simulink library "Simple_lib"  (R2018b)
settings: Solver=ode45  StartTime=0.0  StopTime=10.0  RelTol=1e-3  EnableMultiTasking=on
undefined symbols (not defined in the file or in its folder): Acceptance, beta, C, C_J, C_P, c_wall, dGain, DiscIntNeverNeededParam, Duplex, Electrical_lib, grab, h_fe, i, i3, K_T, Kman, KmanCE, mu_s, n_rev, R_arm, Simplex, systemTs, tau_0, TinIC, Ts, w_0, wallMass, Watch_lib
libraries: $bdroot x407, PlantUtilityBlockset_lib x30, peGeneralControl x22, simulink x11
(part 3 of 14)

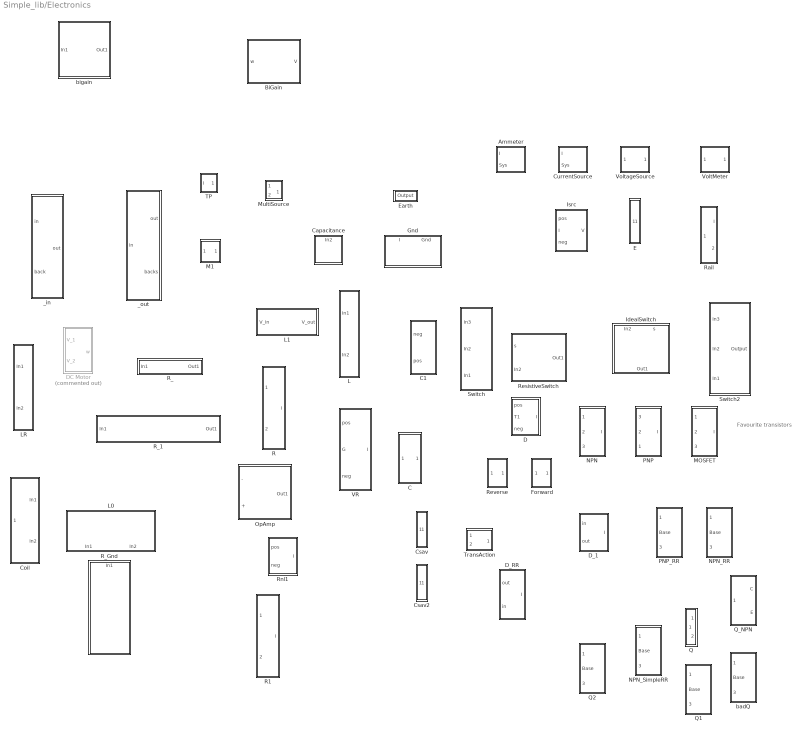
== system Simple_lib/Electronics ==
  note: Favourite transistors
  Ammeter : Subsystem
      mask Display:
      | color('blue')
      | %plot([-1 -.9 -.5 0 .5 .9 1  .9  .5  0 -.5 -.9 -1],      [ 0  .5 .9 1 .9 .5 0 -.5 -.9 -1 -.9 -.5  0]);
      | patch([-1 -.9 -.5 0 .5 .9 1],  [ 0  .5 .9 1 .9 .5 0], [0 0 1]);
      | 
      | %patch([1  .9  .5  0 -.5 -.9 -1], [ 0 -.5 -.9 -1 -.9 -.5  0], [0 0 0]);
      | plot([1  .9  .5  0 -.5 -.9 -1], [ 0 -.5 -.9 -1 -.9 -.5  0]);
      | color('black')
      | disp('A')
      | %plot([0.2 0 -0.2], -[0.7 0.8 0.7])
      | %color('black')
      | %plot([0 0], [0.8 -0.8])
      | 
      | %port_label('output', 1, 'sys ')
      | %color('black')
      | %port_label('output', 2, 'sim ')
  BiGain : Subsystem  mask{k_level=-1, k_flow=-1}
      mask prompts: k_level "Potential Gain"; k_flow "Flow Gain"
      settings: AttributesFormatString="%<k_flow>   %<k_level>"
      mask Display:
      | patch( [0 1 0],[1 0 -1])
      | color('green')
      | plot( [0 -1 0],[1 0 -1])
  C : Subsystem  mask{C=100e-6, Q_0=0}
      mask prompts: C "Capacitance"; Q_0 "Initial Charge (C)"
      settings: AttributesFormatString=%<C>F
      mask Display:
      | %plot([1.0 1.8 1.8 1.0], [0 .1 -.1 0])
      | %patch([-1 -1 -.7 -.7 -1], [-1 1 1 -1 -1])
      | %patch([1 1 .7 .7 1], [-1 1 1 -1 -1])
      | plot([-1 -1], [-1 1])
      | plot([1 1], [-1 1])
      | color('white')
      | plot([-1.1 -1.1], [-1 1])
      | plot([1.1 1.1], [-1 1])
  C1 : Subsystem  mask{C=100e-6}
      mask prompts: C "Capacitance"
      settings: AttributesFormatString=%<C> F
      mask Display:
      | plot([-1 1], [0.5 0.5])
      | plot([-1 1], [-0.5 -0.5])
      | 
      | 
      | color('white')
      | plot([-1 1 1 -1 -1], [-1 -1 1 1 -1])
  Capacitance : Subsystem  mask{C=1e-6}
      mask prompts: C "Capacitance with ground (F)"
      settings: AttributesFormatString=%<C> F
      mask Display:
      | %plot([1.0 1.18 1.18 1.0], [0 .15 -.15 0])
      | plot([0 0],[-1 1])
      | plot([-0.4 -0.4],[-1 1])
      | plot([0.6 0.6], [-0.6 0.6])
      | plot([0.8 0.8],[-0.2 0.2])
      | 
      | plot([-0.4 -1], [0 0])
      | plot([0 0.6],[0 0])
      | 
      | color('white')
      | plot([-1 1 1 -1 -1], [-1 -1 1 1 -1])
  Coil : Subsystem  mask{L=3e-1, R=3e-1, Phi_0=0, L_min=0}
      mask prompts: L "Inductance (H)"; R "Resistance (Ohms)"; Phi_0 "Phi_0 (Vs)"; L_min "L_min (H)"
      settings: AttributesFormatString=|
      | %<L> H
      | %<R> Ohm
      mask Display:
      | %color('black')
      | %plot(   [    0     0.3827     0.7071     0.9239     1.0000     0.9239     0.7071     0.3827     0.0000    -0.3827    -0.7071    -0.9239    -1.0000    -0.9239    -0.7071    -0.3827    -0.0000     0.3827     0.7071     0.9239     1.0000     0.9239     0.7071     0.3827     0.0000    -0.3827    -0.7071    -0.9239    -1.0000    -0.9239    -0.7071    -0.3827    -0.0000     0.3827     0.7071     0.9239     1.0000     0.9239     0.7071     0.3827     0.0000    -0.3827    -0.7071    -0.9239    -1.0000    -0.9239    -0.7071    -0.3827    -0.0000     0.3827     0.7071     0.9239     1.0000     0.9239     0.7071     0.3827     0.0000    -0.3827    -0.7071    -0.9239    -1.0000    -0.9239    -0.7071    -0.3827    -0.0000],   -.5+[-0.0625    -0.0421    -0.0129     0.0230     0.0625     0.1020     0.1379     0.1671     0.1875     0.1984     0.2004     0.1958     0.1875     0.1792     0.1746     0.1766     0.1875     0.2079     0.2371     0.2730     0.3125     0.3520     0.3879     0.4171     0.4375     0.4484     0.4504     0.4458     0.4375     0.4292     0.4246     0.4266     0.4375     0.4579     0.4871     0.5230     0.5625     0.6020     0.6379     0.6671     0.6875     0.6984     0.7004     0.6958     0.6875     0.6792     0.6746     0.6766     0.6875     0.7079     0.7371     0.7730     0.8125     0.8520     0.8879     0.9171     0.9375     0.9484     0.9504     0.9458     0.9375     0.9292     0.9246     0.9266     0.9375])
      | %color('white')
      | %plot([-1 1], [-1 -1])
      | %plot([-1 1], [1 1])
      | color('blue')
      | plot(   .4*[    0     0.3827     0.7071     0.9239     1.0000     0.9239     0.7071     0.3827     0.0000    -0.3827    -0.7071    -0.9239    -1.0000    -0.9239    -0.7071    -0.3827    -0.0000     0.3827     0.7071     0.9239     1.0000     0.9239     0.7071     0.3827     0.0000    -0.3827    -0.7071    -0.9239    -1.0000    -0.9239    -0.7071    -0.3827    -0.0000     0.3827     0.7071     0.9239     1.0000     0.9239     0.7071     0.3827     0.0000    -0.3827    -0.7071    -0.9239    -1.0000    -0.9239    -0.7071    -0.3827    -0.0000     0.3827     0.7071     0.9239     1.0000     0.9239     0.7071     0.3827     0.0000    -0.3827    -0.7071    -0.9239    -1.0000    -0.9239    -0.7071    -0.3827    -0.0000],   -.5+[-0.0625    -0.0421    -0.0129     0.0230     0.0625     0.1020     0.1379     0.1671     0.1875     0.1984     0.2004     0.1958     0.1875     0.1792     0.1746     0.1766     0.1875     0.2079     0.2371     0.2730     0.3125     0.3520     0.3879     0.4171     0.4375     0.4484     0.4504     0.4458     0.4375     0.4292     0.4246     0.4266     0.4375     0.4579     0.4871     0.5230     0.5625     0.6020     0.6379     0.6671     0.6875     0.6984     0.7004     0.6958     0.6875     0.6792     0.6746     0.6766     0.6875     0.7079     0.7371     0.7730     0.8125     0.8520     0.8879     0.9171     0.9375     0.9484     0.9504     0.9458     0.9375     0.9292     0.9246     0.9266     0.9375])
      | plot( [ -.4 .6 -.8 1 ],-.5+[-3:0]/6)
      | plot( [ -.4 .6 -.8 1 ],.5+[0:3]/6)
      | color('white')
      | plot([-1 1 1 -1], [-2 -1 1 2])
  Csav : Subsystem  mask{C=.01, Q_0=0}
      mask prompts: C "Capacitance"; Q_0 "Initial Charge (C)"
      settings: AttributesFormatString=%<C>F
      mask Display:
      | %plot([1.0 1.8 1.8 1.0], [0 .1 -.1 0])
      | %patch([-1 -1 -.7 -.7 -1], [-1 1 1 -1 -1])
      | %patch([1 1 .7 .7 1], [-1 1 1 -1 -1])
      | plot([-1 -1], [-1 1])
      | plot([1 1], [-1 1])
      | color('white')
      | plot([-1.1 -1.1], [-1 1])
      | plot([1.1 1.1], [-1 1])
  Csav2 : Subsystem  mask{C=.01, Q_0=0}
      mask prompts: C "Capacitance"; Q_0 "Initial Charge (C)"
      settings: AttributesFormatString=%<C>F
      mask Display:
      | %plot([1.0 1.8 1.8 1.0], [0 .1 -.1 0])
      | %patch([-1 -1 -.7 -.7 -1], [-1 1 1 -1 -1])
      | %patch([1 1 .7 .7 1], [-1 1 1 -1 -1])
      | plot([-1 -1], [-1 1])
      | plot([1 1], [-1 1])
      | color('white')
      | plot([-1.1 -1.1], [-1 1])
      | plot([1.1 1.1], [-1 1])
  CurrentSource : Subsystem
      mask Display:
      | %plot([-1 -.9 -.5 0 .5 .9 1  .9  .5  0 -.5 -.9 -1],      [ 0  .5 .9 1 .9 .5 0 -.5 -.9 -1 -.9 -.5  0]);
      | 
      | color('blue')
      | %plot([-1 -.9 -.5 0 .5 .9 1  .9  .5  0 -.5 -.9 -1],      [ 0  .5 .9 1 .9 .5 0 -.5 -.9 -1 -.9 -.5  0]);
      | patch([1  .9  .5  0 -.5 -.9 -1],      [ 0 -.5 -.9 -1 -.9 -.5  0], [0 0 1]);
      | 
      | 
      | color('black')
      | plot([-1 -.9 -.5 0 .5 .9 1],      [ 0  .5 .9 1 .9 .5 0]);
      | plot([0 0], [0.8 0])
      | color('white')
      | plot([0 0], [0 -0.8])
      | plot([0.2 0 -0.2], -[0.7 0.8 0.7])
  D : Subsystem  mask{I_S=1e-12, n=2, T_def=300}
      mask prompts: T_def "Default Temp (K)"
      mask Display:
      | %plot( [ -1 0 0 ],[-1 -1 -0.3 ])
      | %plot( [ 0 0 -1],[ 0.3 1 1])
      | plot( [ -1 1],-[1 1]*1.3)
      | plot([-1 1 0 -1],[1 1 -1 1]*1.3)
      | color('white')
      | plot([-1 1], [-2 -2])
      | plot([-1 1], [2 2])
      | %port_label('input', 1, '1')
  DC Motor : Subsystem  Commented=on  mask{k_flow=1, J_mot=1e-3, R_arm=2.0}
      mask prompts: k_flow "Torque constant (Nm/A)"; J_mot "Intertia  (kgm^2)"; R_arm "Armature resistance (Ohm)"
      mask Display:
      | %color('black')
      | %plot( [ -1 0  ],[-1 -1 ])
      | %plot( [ -1 0 ],[ 1 1])
      | 
      | plot([-1 -.9 -.5 0 .5 .9 1  .9  .5  0 -.5 -.9 -1],      [ 0  .5 .9 1 .9 .5 0 -.5 -.9 -1 -.9 -.5  0]);
      | %patch([0 1 1 0 0]-.5,[0 0 1 1 0]*.5-1.5,[0,0,1])
      | %patch([0 1 1 0 0]-.5,[0 0 1 1 0]*.5+1,[0,0,1])
      | color('blue')
      | plot([0 1 1 0 0]-.5,[0 0 1 1 0]*.5-1.5)
      | plot([0 1 1 0 0]-.5,[0 0 1 1 0]*.5+1)
      | %port_label('input', 1, '+')
      | %port_label('input', 2, '-')
      | %port_label('output', 1, 'V')
      | %color('white')
      | %plot([-1 1 1 -1 -1], [-1 -1 1 1 -1]*2)
  D_1 : Subsystem  mask{g_on=0.001, g_off=1e-5, V_drop=1.4}
      mask prompts: g_on "On Conductance (Siemens)"; g_off "Off Conductance (Siemens)"; V_drop "Voltage drop (V)"
      mask Display:
      | %plot( [ -1 0 0 ],[-1 -1 -0.3 ])
      | %plot( [ 0 0 -1],[ 0.3 1 1])
      | plot( [ -1 1],-[1 1]*1.3)
      | patch([-1 1 0 -1],[1 1 -1 1]*1.3)
      | color('white')
      | plot([-1 1], [-2 -2])
      | plot([-1 1], [2 2])
      | %port_label('input', 1, '1')
  D_RR : Subsystem  mask{g=1e-3, V_drop=0.6}
      mask prompts: g "Conductance (Siemens)"; V_drop "Voltage drop (V)"
      mask Display:
      | %plot( [ -1 0 0 ],[-1 -1 -0.3 ])
      | %plot( [ 0 0 -1],[ 0.3 1 1])
      | plot( [ -1 1],-[1 1]*1.3)
      | plot([-1 1 0 -1],[1 1 -1 1]*1.3)
      | color('white')
      | plot([-1 1], [-2 -2])
      | plot([-1 1], [2 2])
      | %port_label('input', 1, '1')
  E : Subsystem  mask{Vbatt=0}
      mask prompts: Vbatt "Voltage (V)"
      settings: AttributesFormatString=EMF: %<Vbatt> V
      mask Display:
      | %color('black')
      | plot([-1 -1], [-0.5 0.5])
      | plot([1 1], [-1 1.0])
      | plot([1 1.1], [0 0])
      | %color('white')
      | %plot([-1 1 1 -1 -1], [-1 -1 1 1 -1])
  Earth : Subsystem
      mask Display:
      | plot([-0.4 -0.4],[-1 1])
      | plot([-0.6 -0.6], [-0.6 0.6])
      | plot([-0.8 -0.8],[-0.2 0.2])
  Forward : Subsystem  mask{V_drop=0.6}
      mask prompts: V_drop "Potential Drop (V)"
      mask Display:
      | patch( [1 1.05 1.05 1],[-1 -1 1 1])
      | patch( [1 0 0],[0 1 -1])
  Gnd : Subsystem
      mask Display:
      | %color('black')
      | %plot([1.0 1.18 1.18 1.0], [0 .15 -.15 0])
      | 
      | plot([-0.1 -0.1],[-.7 .8]+.4)
      | plot([-0.3 -0.3], [-0.6 0.6]+.5)
      | plot([-0.5 -0.5],[-0.2 0.2]+.5)
      | 
      | %plot([-0.1 -0.5],[-1.5 -1.5])
      | 
      | plot([-1 -.9 -.5 0 .5 .9 1  .9  .5  0 -.5 -.9 -1]*.4-.5,      [ 0  .5 .9 1 .9 .5 0 -.5 -.9 -1 -.9 -.5  0]*.9-1.2);
      | plot([-.6 -.3 -.6],[0 .2 .4]-1.3)
      | plot([-.5 -.5],[.1 .3]-1.3)
      | %fprintf('A')
      | %disp('A')
      | %color('white')
      | %plot([-1 1 1 -1 -1], [-1 -1 1 1 -1])
  IdealSwitch : Subsystem
      mask Display:
      | %color('black')
      | %plot([1.0 1.18 1.18 1.0], [0 .2 -.2 0])
      | plot([-1 -0.5], [-0.66 -0.35])
      | plot([-1.0 -0.5]+.3, [-0.66 -0.35]+.5)
      | plot([-.75 -0.5]+.6, [-0.5 -0.35]+.35)
      | 
      | plot([0.1 1], [0 0])
      | plot([-1 -0.5], [0.65 0])
      | color('white')
      | plot([-1 1 1 -1 -1], [-1 -1 1 1 -1])
  Isrc : Subsystem
      mask Display:
      | plot( [ .2 0 -.2],[ -0.4 -.5 -.4])
      | plot( [ 0 0 ],[-1 1]*.5)
      | plot([-1 0 1 0 -1],[0 0.7 0 -0.7 0])
      | port_label('input', 1, '+')
      | port_label('input', 3, '-')
      | color('black')
      | port_label('output', 1, 'V ')
      | port_label('input', 2, ' I')
      | 
      | 
      | color('white')
      | plot([-1 1],[-1 -1])
      | plot([-1 1],[1 1])
  L : Subsystem  mask{L=.1, V_0=0}
      mask prompts: L "Inductance (H)"; V_0 "Initial field"
      settings: AttributesFormatString=|
      | %<L> H
      | %<V_0>
      mask Display:
      | %color('black')
      | plot(   [    0     0.3827     0.7071     0.9239     1.0000     0.9239     0.7071     0.3827     0.0000    -0.3827    -0.7071    -0.9239    -1.0000    -0.9239    -0.7071    -0.3827    -0.0000     0.3827     0.7071     0.9239     1.0000     0.9239     0.7071     0.3827     0.0000    -0.3827    -0.7071    -0.9239    -1.0000    -0.9239    -0.7071    -0.3827    -0.0000     0.3827     0.7071     0.9239     1.0000     0.9239     0.7071     0.3827     0.0000    -0.3827    -0.7071    -0.9239    -1.0000    -0.9239    -0.7071    -0.3827    -0.0000     0.3827     0.7071     0.9239     1.0000     0.9239     0.7071     0.3827     0.0000    -0.3827    -0.7071    -0.9239    -1.0000    -0.9239    -0.7071    -0.3827    -0.0000],   -.5+[-0.0625    -0.0421    -0.0129     0.0230     0.0625     0.1020     0.1379     0.1671     0.1875     0.1984     0.2004     0.1958     0.1875     0.1792     0.1746     0.1766     0.1875     0.2079     0.2371     0.2730     0.3125     0.3520     0.3879     0.4171     0.4375     0.4484     0.4504     0.4458     0.4375     0.4292     0.4246     0.4266     0.4375     0.4579     0.4871     0.5230     0.5625     0.6020     0.6379     0.6671     0.6875     0.6984     0.7004     0.6958     0.6875     0.6792     0.6746     0.6766     0.6875     0.7079     0.7371     0.7730     0.8125     0.8520     0.8879     0.9171     0.9375     0.9484     0.9504     0.9458     0.9375     0.9292     0.9246     0.9266     0.9375])
      | color('white')
      | plot([-1 1], [-1 -1])
      | plot([-1 1], [1 1])
  L0 : Subsystem  mask{L=.1, R=1e3}
      mask prompts: L "Inductance (H)"; R "Resistance (Ohms)"
      settings: AttributesFormatString=|
      | %<L> H
      | %<R> Ohm
      mask Display:
      | %color('black')
      | plot(   [    0     0.3827     0.7071     0.9239     1.0000     0.9239     0.7071     0.3827     0.0000    -0.3827    -0.7071    -0.9239    -1.0000    -0.9239    -0.7071    -0.3827    -0.0000     0.3827     0.7071     0.9239     1.0000     0.9239     0.7071     0.3827     0.0000    -0.3827    -0.7071    -0.9239    -1.0000    -0.9239    -0.7071    -0.3827    -0.0000     0.3827     0.7071     0.9239     1.0000     0.9239     0.7071     0.3827     0.0000    -0.3827    -0.7071    -0.9239    -1.0000    -0.9239    -0.7071    -0.3827    -0.0000     0.3827     0.7071     0.9239     1.0000     0.9239     0.7071     0.3827     0.0000    -0.3827    -0.7071    -0.9239    -1.0000    -0.9239    -0.7071    -0.3827    -0.0000],   -.5+[-0.0625    -0.0421    -0.0129     0.0230     0.0625     0.1020     0.1379     0.1671     0.1875     0.1984     0.2004     0.1958     0.1875     0.1792     0.1746     0.1766     0.1875     0.2079     0.2371     0.2730     0.3125     0.3520     0.3879     0.4171     0.4375     0.4484     0.4504     0.4458     0.4375     0.4292     0.4246     0.4266     0.4375     0.4579     0.4871     0.5230     0.5625     0.6020     0.6379     0.6671     0.6875     0.6984     0.7004     0.6958     0.6875     0.6792     0.6746     0.6766     0.6875     0.7079     0.7371     0.7730     0.8125     0.8520     0.8879     0.9171     0.9375     0.9484     0.9504     0.9458     0.9375     0.9292     0.9246     0.9266     0.9375])
      | color('white')
      | plot([-1 1], [-1 -1])
      | plot([-1 1], [1 1])
  L1 : Subsystem  mask{L=1, R=0}
      mask prompts: L "Inductance (H)"; R "Resistance (Ohms)"
      settings: AttributesFormatString=|
      | %<L> H
      | %<R> Ohm
      mask Display:
      | %color('white')
      | %plot([-1 1 1 -1 -1], [-1 -1 1 1 -1])
      | %color('black')
      | %plot([1.0 1.18 1.18 1.0], [0 .2 -.2 0])
      | plot(-1+2*[-0.0625
      |    -0.0421
      |    -0.0129
      |     0.0230
      |     0.0625
      |     0.1020
      |     0.1379
      |     0.1671
      |     0.1875
      |     0.1984
      |     0.2004
      |     0.1958
      |     0.1875
      |     0.1792
      |     0.1746
      |     0.1766
      |     0.1875
      |     0.2079
      |     0.2371
      |     0.2730
      |     0.3125
      |     0.3520
      |     0.3879
      |     0.4171
      |     0.4375
      |     0.4484
      |     0.4504
      |     0.4458
      |     0.4375
      |     0.4292
      |     0.4246
      |     0.4266
      |     0.4375
      |     0.4579
      |     0.4871
      |     0.5230
      |     0.5625
      |     0.6020
      |     0.6379
      |     0.6671
      |     0.6875
      |     0.6984
      |     0.7004
      |     0.6958
      |     0.6875
      |     0.6792
      |     0.6746
      |     0.6766
      |     0.6875
      |     0.7079
      |     0.7371
      |     0.7730
      |     0.8125
      |     0.8520
      |     0.8879
      |     0.9171
      |     0.9375
      |     0.9484
      |     0.9504
      |     0.9458
      |     0.9375
      |     0.9292
      |     0.9246
      |     0.9266
      |     0.9375], [    0
      |     0.3827
      |     0.7071
      |     0.9239
      |     1.0000
      |     0.9239
      |     0.7071
      |     0.3827
      |     0.0000
      |    -0.3827
      |    -0.7071
      |    -0.9239
      |    -1.0000
      |    -0.9239
      |    -0.7071
      |    -0.3827
      |    -0.0000
      |     0.3827
      |     0.7071
      |     0.9239
      |     1.0000
      |     0.9239
      |     0.7071
      |     0.3827
      |     0.0000
      |    -0.3827
      |    -0.7071
      |    -0.9239
      |    -1.0000
      |    -0.9239
      |    -0.7071
      |    -0.3827
      |    -0.0000
      |     0.3827
      |     0.7071
      |     0.9239
      |     1.0000
      |     0.9239
      |     0.7071
      |     0.3827
      |     0.0000
      |    -0.3827
      |    -0.7071
      |    -0.9239
      |    -1.0000
      |    -0.9239
      |    -0.7071
      |    -0.3827
      |    -0.0000
      |     0.3827
      |     0.7071
      |     0.9239
      |     1.0000
      |     0.9239
      |     0.7071
      |     0.3827
      |     0.0000
      |    -0.3827
      |    -0.7071
      |    -0.9239
      |    -1.0000
      |    -0.9239
      |    -0.7071
      |    -0.3827
      |    -0.0000])
  LR : Subsystem  mask{L=1e-6, R=R_arm, Phi_0=0}
      mask prompts: L "Inductance (H)"; R "Resistance (Ohms)"; Phi_0 "Phi_0 (Vs)"
      settings: AttributesFormatString=|
      | %<L> H
      | %<R> Ohm
      mask Display:
      | %color('black')
      | %plot(   [    0     0.3827     0.7071     0.9239     1.0000     0.9239     0.7071     0.3827     0.0000    -0.3827    -0.7071    -0.9239    -1.0000    -0.9239    -0.7071    -0.3827    -0.0000     0.3827     0.7071     0.9239     1.0000     0.9239     0.7071     0.3827     0.0000    -0.3827    -0.7071    -0.9239    -1.0000    -0.9239    -0.7071    -0.3827    -0.0000     0.3827     0.7071     0.9239     1.0000     0.9239     0.7071     0.3827     0.0000    -0.3827    -0.7071    -0.9239    -1.0000    -0.9239    -0.7071    -0.3827    -0.0000     0.3827     0.7071     0.9239     1.0000     0.9239     0.7071     0.3827     0.0000    -0.3827    -0.7071    -0.9239    -1.0000    -0.9239    -0.7071    -0.3827    -0.0000],   -.5+[-0.0625    -0.0421    -0.0129     0.0230     0.0625     0.1020     0.1379     0.1671     0.1875     0.1984     0.2004     0.1958     0.1875     0.1792     0.1746     0.1766     0.1875     0.2079     0.2371     0.2730     0.3125     0.3520     0.3879     0.4171     0.4375     0.4484     0.4504     0.4458     0.4375     0.4292     0.4246     0.4266     0.4375     0.4579     0.4871     0.5230     0.5625     0.6020     0.6379     0.6671     0.6875     0.6984     0.7004     0.6958     0.6875     0.6792     0.6746     0.6766     0.6875     0.7079     0.7371     0.7730     0.8125     0.8520     0.8879     0.9171     0.9375     0.9484     0.9504     0.9458     0.9375     0.9292     0.9246     0.9266     0.9375])
      | %color('white')
      | %plot([-1 1], [-1 -1])
      | %plot([-1 1], [1 1])
      | 
      | plot(   .4*[    0     0.3827     0.7071     0.9239     1.0000     0.9239     0.7071     0.3827     0.0000    -0.3827    -0.7071    -0.9239    -1.0000    -0.9239    -0.7071    -0.3827    -0.0000     0.3827     0.7071     0.9239     1.0000     0.9239     0.7071     0.3827     0.0000    -0.3827    -0.7071    -0.9239    -1.0000    -0.9239    -0.7071    -0.3827    -0.0000     0.3827     0.7071     0.9239     1.0000     0.9239     0.7071     0.3827     0.0000    -0.3827    -0.7071    -0.9239    -1.0000    -0.9239    -0.7071    -0.3827    -0.0000     0.3827     0.7071     0.9239     1.0000     0.9239     0.7071     0.3827     0.0000    -0.3827    -0.7071    -0.9239    -1.0000    -0.9239    -0.7071    -0.3827    -0.0000],   -.5+[-0.0625    -0.0421    -0.0129     0.0230     0.0625     0.1020     0.1379     0.1671     0.1875     0.1984     0.2004     0.1958     0.1875     0.1792     0.1746     0.1766     0.1875     0.2079     0.2371     0.2730     0.3125     0.3520     0.3879     0.4171     0.4375     0.4484     0.4504     0.4458     0.4375     0.4292     0.4246     0.4266     0.4375     0.4579     0.4871     0.5230     0.5625     0.6020     0.6379     0.6671     0.6875     0.6984     0.7004     0.6958     0.6875     0.6792     0.6746     0.6766     0.6875     0.7079     0.7371     0.7730     0.8125     0.8520     0.8879     0.9171     0.9375     0.9484     0.9504     0.9458     0.9375     0.9292     0.9246     0.9266     0.9375])
      | plot( [ -.4 .6 -.8 1 ],-.5+[-3:0]/6)
      | plot( [ -.4 .6 -.8 1 ],.5+[0:3]/6)
      | color('white')
      | plot([-1 1 1 -1], [-2 -1 1 2])
  M1 : Subsystem
      mask Display:
      | plot([-1 -.9 -.5 0 .5 .9 1  .9  .5  0 -.5 -.9 -1],      [ 0  .5 .9 1 .9 .5 0 -.5 -.9 -1 -.9 -.5  0]);
      | disp('M')
  MOSFET : Subsystem  mask{V_T=1.7, k=5}
      mask Display:
      | patch([0 0 0.05 0.05]-0.2,[-.3 .3 .3 -.3])
      | patch([0 0 0.1 0.1],[-1 1 1 -1])
      | %patch([0 0 0.1 0.1],[-1 -.6 -.6 -1],[.9 .5 .1])
      | 
      | plot([0 1],[0.66 0.66])
      | plot([0 1],[0 0])
      | plot([0 1],[-0.66 -0.66])
      | plot([1 1],[-0.66 0])
      | patch([0.1 .3 .3],[0 .1 -0.1])
  MultiSource : Subsystem  mask{V_0=inf, slew_rate=inf, conserved_quantity_name=Q, energy_name=E}
      mask prompts: V_0 "Iniitial Potential (V)"; slew_rate "Max +/- slew rate (V/s)"; conserved_quantity_name "Conserved quantity name"; energy_name "Energy name"
      mask init:
      | init_lump
      mask Display:
      | plot([-1 -.9 -.5 0 .5 .9 1  .9  .5  0 -.5 -.9 -1],      [ 0  .5 .9 1 .9 .5 0 -.5 -.9 -1 -.9 -.5  0]);
      | %disp(get(gcbh,'Name'))
  NPN : Subsystem  mask{alpha_F=0.98, alpha_R=0.9, n=1, I_S=1e-12, T_def=300}
      mask prompts: n "Emission Coefficient"; T_def "Default temp (when input==0) (K)"
      mask Display:
      | patch([0 0 0.1 0.1],[-1 1 1 -1])
      | %patch([0 0 0.1 0.1],[-1 -.7 -.7 -1],[.9 .5 .1])
      | 
      | plot([0 1],[0.25 1])
      | plot([0 1],[-0.25 -1])
      | 
      | patch([.8 1 1],[-1 -1 -0.8])
  NPN_RR : Subsystem  mask{alpha_F=0.98, alpha_R=0.9}
      mask Display:
      | patch([0 0 0.1 0.1],[-1 1 1 -1])
      | %patch([0 0 0.1 0.1],[-1 -.7 -.7 -1],[.9 .5 .1])
      | 
      | plot([0 1],[0.25 1])
      | plot([0 1],[-0.25 -1])
      | 
      | patch([.8 1 1],[-1 -1 -0.8])
  NPN_SimpleRR : Subsystem  mask{alpha_F=0.98, alpha_R=0.9}
      mask Display:
      | patch([0 0 0.1 0.1],[-1 1 1 -1])
      | %patch([0 0 0.1 0.1],[-1 -.7 -.7 -1],[.9 .5 .1])
      | 
      | plot([0 1],[0.25 1])
      | plot([0 1],[-0.25 -1])
      | 
      | patch([.8 1 1],[-1 -1 -0.8])
  OpAmp : Subsystem  mask{K_op=6}
      mask prompts: K_op "K_op (-)"
      mask Display:
      | %patch( [1 1.05 1.05 1],[-1 -1 1 1])
      | plot( [1 0 0 1],[0 1 -1 0])
      | port_label('input', 1, '+')
      | port_label('input', 2, '-')
  PNP : Subsystem  mask{alpha_F=0.98, alpha_R=0.9}
      mask Display:
      | patch([0 0 0.1 0.1],[-1 1 1 -1])
      | %patch([0 0 0.1 0.1],[-1 -.7 -.7 -1],[.9 .5 .1])
      | 
      | plot([0 1],[0.25 1])
      | plot([0 1],[-0.25 -1])
      | 
      | patch([.1 .35 .2],[-0.25 -0.35 -0.5])
  PNP_RR : Subsystem  mask{alpha_F=0.98, alpha_R=0.9}
      mask Display:
      | patch([0 0 0.1 0.1],[-1 1 1 -1])
      | %patch([0 0 0.1 0.1],[-1 -.7 -.7 -1],[.9 .5 .1])
      | 
      | plot([0 1],[0.25 1])
      | plot([0 1],[-0.25 -1])
      | 
      | patch([.1 .35 .2],[-0.25 -0.35 -0.5])
  Q : Subsystem  mask{alpha_F=0.98, alpha_R=0.9}
      mask Display:
      | patch([1 1 0.9 0.9],[-1 1 1 -1])
      | %patch([0 0 0.1 0.1],[-1 -.7 -.7 -1],[.9 .5 .1])
      | 
      | plot([1 0], [0.05 0.5])
      | plot([1 0], [-0.05 -0.5])
      | 
      | patch([.2 0 0.1], [-.5 -.5 -0.35])
  Q1 : Subsystem  mask{alpha_F=0.98, alpha_R=0.9, g_on=10, g_off=1e-6, V_drop=0.6}
      mask prompts: g_on "diode g on (S)"; g_off "diode g off"; V_drop "diode drop (V)"
      mask Display:
      | patch([0 0 0.1 0.1],[-1 1 1 -1])
      | %patch([0 0 0.1 0.1],[-1 -.7 -.7 -1],[.9 .5 .1])
      | 
      | plot([0 1],[0.25 1])
      | plot([0 1],[-0.25 -1])
      | 
      | patch([.8 1 1],[-1 -1 -0.8])
  Q2 : Subsystem  mask{alpha_F=0.98, alpha_R=0.9, g_on=10, g_off=1e-6, V_drop=0.6}
      mask Display:
      | patch([0 0 0.1 0.1],[-1 1 1 -1])
      | %patch([0 0 0.1 0.1],[-1 -.7 -.7 -1],[.9 .5 .1])
      | 
      | plot([0 1],[0.25 1])
      | plot([0 1],[-0.25 -1])
      | 
      | patch([.1 .35 .2],[-0.25 -0.35 -0.5])
  Q_NPN : Subsystem  mask{alpha_F=0.98, alpha_R=0.1}
      mask Display:
      | patch([0 0 0.1 0.1],0.5*[-1 1 1 -1])
      | %patch([0 0 0.1 0.1],[-1 -.7 -.7 -1],[.9 .5 .1])
      | 
      | plot([0 1],[0.2 0.5])
      | plot([0 1],[-0.2 -0.5])
      | 
      | patch([.8 1 1],[-0.53 -0.53 -0.4])
      | color('white')
      | plot([0 0],[-1 1])
  R : Subsystem  mask{R=100e3}
      mask prompts: R "Resistance (Ohms)"
      settings: AttributesFormatString=%<R> Ohms
      mask Display:
      | plot( [ -1 1 -1 1 -1 1 -1],[-3:3]/6)
      | 
      | port_label('input',1,'+')
      | port_label('input',2,'-')
      | color('white')
      | plot([-1 1 1 -1 -1], [-1 -1 1 1 -1])
  R1 : Subsystem  mask{R=100e3}
      mask prompts: R "Resistance (Ohms)"
      settings: AttributesFormatString=%<R> Ohms
      mask Display:
      | plot( [ -1 1 -1 1 -1 1 -1],[-3:3]/6)
      | 
      | port_label('input',1,'+')
      | port_label('input',2,'-')
      | color('white')
      | plot([-1 1 1 -1 -1], [-1 -1 1 1 -1])
  R_ : Subsystem  mask(Circuit Resistor){Mantissa=1.0, Exponent=3, R=1000}
      mask prompts: Mantissa "Resistance (Ohm)"; Exponent "e"
      mask help: This block contains an Ohmic Resistance, and a test point at its outport.
      mask init:
      | newR = str2num(Mantissa) * 10^Exponent;
      | set(gcbh,'R', num2str(newR))
      settings: AttributesFormatString=%<R> Ohm
      mask Help:
      | Choose one of the standard resistance values or type your own.
      | e means the power of 10 that the chosen resistance value will be multiplied by to make the actual resistance used.
      mask TypeOptions Mantissa: 1.0 | 1.2 | 1.5 | 1.8 | 2.2 | 2.7 | 3.3 | 3.9 | 4.7 | 5.6 | 6.8 | 8.2
      mask DialogControl Exponent Tooltip: Times this power of ten
      mask Display:
      | %color('black')
      | %plot([1.0 1.18 1.18 1.0], [0 .2 -.2 0])
      | plot([-8:8]/8, [0 1 0 -1 0 1 0 -1 0 1 0 -1 0 1 0 -1 0])
      | 
      | color('white')
      | plot([-1 1 1 -1 -1], [-1 -1 1 1 -1])
  R_1 : Subsystem  mask{R=0}
      mask prompts: R "Resistance"
      settings: AttributesFormatString=%<R> Ohm
      mask Display:
      | %color('black')
      | %plot([1.0 1.18 1.18 1.0], [0 .2 -.2 0])
      | plot([-8:8]/8, [0 1 0 -1 0 1 0 -1 0 1 0 -1 0 1 0 -1 0])
      | 
      | color('white')
      | plot([-1 1 1 -1 -1], [-1 -1 1 1 -1])
  R_Gnd : Subsystem  mask{R=15e3}
      mask prompts: R "Resistance"
      settings: AttributesFormatString=%<R> Ohm
      mask Display:
      | %color('black')
      | %plot([1.0 1.18 1.18 1.0], [0 .2 -.2 0])
      | plot([-8:8]/8, [0 1 0 -1 0 1 0 -1 0 1 0 -1 0 1 0 -1 0])
      | 
      | plot([0 0]+2.6, 0.9*[-1 1])
      | plot([0 0]+2.8, 0.75*[-1 1])
      | plot([0 0]+3, 0.5*[-1 1])
      | 
      | plot([1 2.6],[0 0])
      | 
      | color('white')
      | plot([-1 1 1 -1 -1], [-1 -1 1 1 -1])
  Rail : Subsystem  mask{Vcc=12}
      mask prompts: Vcc "Vcc offset  (V)"
      settings: AttributesFormatString=in +%<Vcc> V
      mask Display:
      | %color('black')
      | plot([-.9 -.9], [-0.5 0.5])
      | plot([.9 .9], [-1 1.0])
      | color('white')
      | plot([-1 1 1 -1 -1], [-1 -1 1 1 -1])
  ResistiveSwitch : Subsystem
      mask Display:
      | %color('black')
      | %plot([1.0 1.18 1.18 1.0], [0 .2 -.2 0])
      | plot([-1 -0.5], [-0.66 -0.35])
      | plot([-1.0 -0.5]+.3, [-0.66 -0.35]+.5)
      | plot([-.75 -0.5]+.6, [-0.5 -0.35]+.35)
      | 
      | plot([0.1 1], [0 0])
      | plot([-1 -0.5], [0.65 0])
      | color('white')
      | plot([-1 1 1 -1 -1], [-1 -1 1 1 -1])
  Reverse : Subsystem  mask{V_drop=0}
      mask prompts: V_drop "Potential Drop (V)"
      mask Display:
      | patch( [0 -0.05 -0.05 0],[-1 -1 1 1])
      | patch( [0 1 1],[0 1 -1])
  Rnl1 : Subsystem  mask{I_S=1e-12, n=2, T_def=300}
      mask prompts: T_def "Default Temp (K)"
      mask Display: plot( [ -1.2 0.8 -1 1.2 -1 1.5 -1],[-3:3]/6)
  Switch : Subsystem
      mask Display:
      | %color('black')
      | plot( [ -1 0 0 ], [ 1 1 .3 ]*2/3 )
      | plot( [ -1 0 0 ],-[ 1 1 .3 ]*2/3 )
      | plot( [ -1 -1 ]/2,[ -.3 .3 ]*2/3 )
      | 
      | color('white')
      | plot([-1 1 1 -1 -1], [-1 -1 1 1 -1])
  Switch2 : Subsystem
      mask Display:
      | %color('black')
      | plot( [ -1 0 0 ], [ 1 1 .3 ]*2/3 )
      | plot( [ -1 0 0 ],-[ 1 1 .3 ]*2/3 )
      | plot( [ 0 1 ],[ .2 0 ] )
      | patch( [ 0 .22 0],[ .2 .22 .15] )
      | plot( [ -1 +.7 ],[ 0 0 ] )
      | 
      | color('white')
      | plot([-1 1 1 -1 -1], [-1 -1 1 1 -1])
  TP : Subsystem  mask{V_0=0.0, slew_rate=inf, conserved_quantity_name=Q, energy_name=E}
      mask prompts: V_0 "Iniitial Potential (V)"; slew_rate "Max +/- slew rate (V/s)"; conserved_quantity_name "Conserved quantity name"; energy_name "Energy name"
      mask init:
      | init_lump
      mask Display:
      | plot([-1 -.9 -.5 0 .5 .9 1  .9  .5  0 -.5 -.9 -1],      [ 0  .5 .9 1 .9 .5 0 -.5 -.9 -1 -.9 -.5  0]);
      | %disp(get(gcbh,'Name'))
  TransAction : Subsystem  mask{V_drop=.6}
      mask prompts: V_drop "Potential Drop (V)"
      mask Display:
      | patch( [0 -0.05 -0.05 0],[-1 -1 1 1])
      | patch( [0 1 1],[0 1 -1])
  VR : Subsystem
      mask Display:
      | plot( [ -1 1 -1 1 -1 1 -1],[-3:3]/6)
      | plot( [ 1 -1]*0.8,[-1 1]*0.8)
      | patch([0.6 0.8 0.8],-[0.8 0.8 0.6])
      | color('white')
      | plot([-1 1 1 -1 -1], [-1 -1 1 1 -1])
  VoltMeter : Subsystem
      mask Display:
      | %plot([-1 -.9 -.5 0 .5 .9 1  .9  .5  0 -.5 -.9 -1],      [ 0  .5 .9 1 .9 .5 0 -.5 -.9 -1 -.9 -.5  0]);
      | color('black')
      | plot([0 .5 .9 1  .9  .5  0],      [ 1 .9 .5 0 -.5 -.9 -1]);
      | patch(-[0 .5 .9 1  .9  .5  0],  [ 1 .9 .5 0 -.5 -.9 -1] ,[0 0 1]  );
      | %plot([0 0], [0 -0.8])
      | %plot([0.2 0 -0.2], -[0.7 0.8 0.7])
      | %port_label('output', 1, '+ ')
      | color('black')
      | disp('V')
  VoltageSource : Subsystem
      mask Display:
      | %plot([-1 -.9 -.5 0 .5 .9 1  .9  .5  0 -.5 -.9 -1],      [ 0  .5 .9 1 .9 .5 0 -.5 -.9 -1 -.9 -.5  0]);
      | %plot([0 0], [0 -0.8])
      | %plot([0.2 0 -0.2], -[0.7 0.8 0.7])
      | patch([0 .5 .9 1  .9  .5  0],      [ 1 .9 .5 0 -.5 -.9 -1], [0 0 1]);
      | color('black')
      | plot(-[0 .5 .9 1  .9  .5  0],  [ 1 .9 .5 0 -.5 -.9 -1] );
      | %port_label('input', 1, ' V')
      | color('white')
      | port_label('output', 1, '+ ')
  _in : Subsystem  InitFcn=""  mask{Level=V, Flow=I}
      mask prompts: Level "Level variable name:"; Flow "Flow variable name:"
      mask init:
      | init_in
      mask Display:
      | %% Icon for flow in
      | % Signally design
      | %plot([0 2 2 3], [1 1 0 0])
      | %plot([1 3 2 1 0 2], [0.6 0.6 0.4 0.6 0.4 0.4])
      | %patch([1 3 2],[0.6 0.6 0.4])
      | %plot([0 1 1], [1 1 0.6])
      | %plot([1 1 0], [0.4 -1 -1])
      | 
      | %color('white')
      | %plot([0 3], [2 2])
      | %plot([0 3], [-2 -2])
      | 
      | %% Bolder design
      | %patch( [0 1 -1], [0 1 1])
      | %plot( [-1 1], [1.05 1.05])
      | %patch( [-0.1 -0.1 -1], [0.95 0 0.95])
      | patch( [-0.1 -0.1 -1], [1 0 1])
      | patch( [0.1 0.1 1], [1 0 1])
      | plot( [0.1 1 -1 -0.1], [0 -2 -2 0]*0.5)
      | %patch( [-0.1 0.1 0.1 -0.1], [0 0 1 1], [1 1 1])
      | %patch( [-1 0.1 0.1 -1], [1 1 0.95 0.95], [1 1 1])
      | 
      | %% Size the box
      | color('white')
      | plot( [-1 1], [2 2])
      | plot( [-1 1], -[2 2])
  _out : Subsystem  Tag=Electrical  mask{Level=V, Flow=I}
      mask prompts: Level "Level variable name:"; Flow "Flow variable name:"
      mask init:
      | init_out
      mask Display:
      | % This is a new mask on top of the base mask.
      | % Use "View base mask" link below to see the base mask.
      | % Icon for flow out
      | %% Complex icon
      | %plot([0 1 1], [0 0 0.4])
      | %plot([1 1 3], [0.6 1 1])
      | %plot([1 3 2 1 0 2], [0.6 0.6 0.4 0.6 0.4 0.4])
      | %patch([0 2 1],[0.4 0.4 0.6])
      | %plot([3 2 2], [1 1 0.6])
      | %plot([2.2 2.2], [1 0.6])
      | %plot([1.8 1.8], [1 0.6])
      | %plot([1.6 2.4], [0 0])
      | %plot([2 2], [0.1 -0.1])
      | %plot([2 2], [0.4 0.2])
      | %plot([2 2 3], [-0.2 -1 -1])
      | 
      | %color('white')
      | %plot([0 3], [2 2])
      | %plot([0 3], [-2 -2])
      | 
      | %% Bolder icon
      | plot([-1 0 1], [0 -1 0])
      | %patch([-1 1 0 -1], [1 1 2 1]*1-1)
      | patch([-1 -.2 -.2], [0 0 1])
      | patch([1 .2 .2], [0 0 1])
      | %patch( [-0.1 0.1 0.1 -0.1], [0 0 1 1], [1 1 1])
      | plot(0.2*[-1 1],-0.3*[1  1]+0*1.5)
      | plot([0 0],[-0.15 -0.45]+0*1.5)
      | 
      | 
      | color('white')
      | plot( [-1 1], [2 2])
      | plot( [-1 1], -[2 2])
  badQ : Subsystem  mask{alpha_F=0.98, alpha_R=0.9}
      mask Display:
      | patch([0 0 0.1 0.1],[-1 1 1 -1])
      | %patch([0 0 0.1 0.1],[-1 -.7 -.7 -1],[.9 .5 .1])
      | 
      | plot([0 1],[0.25 1])
      | plot([0 1],[-0.25 -1])
      | 
      | patch([.8 1 1],[-1 -1 -0.8])
  bigain : Subsystem
      mask Display:
      | %patch( [1 1.05 1.05 1],[-1 -1 1 1])
      | patch( [1 0 0],[0 1 -1])
      | plot( [0 1 1],[1 2 0])

== system Simple_lib/Hydraulic ==
  " Heat Exchanger" : Subsystem  AncestorBlock="PlantUtilityBlockset_lib/Hydraulic/ Heat  Exchanger"
      mask Display:
      | color('white');
      | plot([-3 3],[1 1]);
      | plot([-3 3],[-1 -1]);
      | color('black')
      | 
      | plot(2+[ 0 .5 .9 1  .9  .5  0 ], [ 1 .9 .5 0 -.5 -.9 -1 ]);
      | plot(-2-[ 0 .5 .9 1  .9  .5  0 ], [ 1 .9 .5 0 -.5 -.9 -1 ]);
      | 
      | plot([-1.5 -1.5],[-1 1]);
      | plot([1.5 1.5],[-1 1]);
      | 
      | plot([-1.5 1.5],[1.0 1.0]);
      | plot([-1.5 1.5],[0.5 0.5]);
      | plot([-1.5 1.5],[0 0]);
      | plot([-1.5 1.5],[-0.5 -0.5]);
      | plot([-1.5 1.5],[-1.0 -1.0]);
  Accumulator : Subsystem
      mask Display:
      | color('white');
      | plot([-1 1],[1 1]);
      | plot([-1 1],[-1 -1]);
      | color('black')
      | plot([0 0],[-1 1]);
      | plot([-1 -.9 -.5 0 .5 .9 1  .9  .5  0 -.5 -.9 -1],      [ 0  .5 .9 1 .9 .5 0 -.5 -.9 -1 -.9 -.5  0]);
      | plot([0 -0.2 -0.4 -0.6],[-0.25 0.25 -0.25 0.25])
      | plot([1 1.5 1.5 1],[0 -0.25 0.25 0])
  Atmosphere : Subsystem
      mask Display:
      | color('white')
      | plot([-1 1 1 -1 -1], [-1 -1 1 1 -1])
      | 
      | color('black')
      | plot([1.0 1.18 1.18 1.0], [0 .15 -.15 0])
      | 
      | plot([-0.4 -0.4],[-1 1])
      | plot([-0.4 0], [-1 -1])
      | plot([-0.4 0],[1 1])
      | 
      | plot([-0.3 1],[0 0])
  Heat Sink : Subsystem
  Isothermal Accumulator : Subsystem
      mask Display:
      | color('white');
      | plot([-1 1],[1 1]);
      | plot([-1 1],[-1 -1]);
      | color('black')
      | plot([0 0],[-1 1]);
      | plot([-1 -.9 -.5 0 .5 .9 1  .9  .5  0 -.5 -.9 -1],      [ 0  .5 .9 1 .9 .5 0 -.5 -.9 -1 -.9 -.5  0]);
      | plot([0 -0.2 -0.4 -0.6],[-0.25 0.25 -0.25 0.25])
      | plot([1 1.5 1.5 1],[0 -0.25 0.25 0])
  Isothermal Pump : Subsystem
      mask Display:
      | color('white');
      | plot([-1 1],[1 1]);
      | plot([-1 1],[-1 -1]);
      | color('black')
      | 
      | plot([-1 -.9 -.5 0 .5 .9 1  .9  .5  0 -.5 -.9 -1],      [ 0  .5 .9 1 .9 .5 0 -.5 -.9 -1 -.9 -.5  0]);
      | 
      | patch([0 -0.25 0.25 0],[1 .5 .5 1])
      | patch([0 -0.25 0.25 0],-[1 .5 .5 1])
  Isothermal Tank : Subsystem
      mask Display:
      | color('white')
      | plot([-1 1 1 -1 -1], [-1 -1 1 1 -1])
      | 
      | color('black')
      | plot([1.0 1.18 1.18 1.0], [0 .15 -.15 0])
      | 
      | plot([-0.4 -0.4],[-1 1])
      | plot([-0.4 0], [-1 -1])
      | plot([-0.4 0],[1 1])
      | 
      | plot([-0.3 1],[0 0])
  Linear Heat Pipe : Subsystem
      mask Display:
      | plot([-1:0.2:1], [1 .8 .6 .5 .5 .5 .5 .5 .6 .8 1])
      | plot([-1:0.2:1], -[1 .8 .6 .5 .5 .5 .5 .5 .6 .8 1])
  Linear Pipe : Subsystem
      mask Display:
      | plot([-1:0.2:1], [1 .8 .6 .5 .5 .5 .5 .5 .6 .8 1])
      | plot([-1:0.2:1], -[1 .8 .6 .5 .5 .5 .5 .5 .6 .8 1])
  Motor : Subsystem
      mask Display:
      | color('white');
      | plot([-1 1],[1 1]);
      | plot([-1 1],[-1 -1]);
      | color('black')
      | 
      | plot([-1 -.9 -.5 0 .5 .9 1  .9  .5  0 -.5 -.9 -1],      [ 0  .5 .9 1 .9 .5 0 -.5 -.9 -1 -.9 -.5  0]);
      | 
      | text(0,0,'M')
      | plot([1 1.5 1.5 1],[0 -0.25 0.25 0])
  Pressure Meter : Subsystem
      mask Display:
      | color('white')
      | plot([-1 1 1 -1 -1], [-1 -1 1 1 -1])
      | color('black')
      | 
      | plot([-1 -.9 -.5 0 .5 .9 1  .9  .5  0 -.5 -.9 -1], ...
      |     [ 0  .5 .9 1 .9 .5 0 -.5 -.9 -1 -.9 -.5  0]);
      | plot(.7*[-1 1], .7*[-1 1])
      | plot(.7*[-1 1], .7*[1 -1])
      | 
      | %text(0, 0, 'p')
  Pump : Subsystem
      mask Display:
      | color('white');
      | plot([-1 1],[1 1]);
      | plot([-1 1],[-1 -1]);
      | color('black')
      | 
      | plot([-1 -.9 -.5 0 .5 .9 1  .9  .5  0 -.5 -.9 -1],      [ 0  .5 .9 1 .9 .5 0 -.5 -.9 -1 -.9 -.5  0]);
      | 
      | patch([0 -0.25 0.25 0],[1 .5 .5 1])
      | patch([0 -0.25 0.25 0],-[1 .5 .5 1])
  Quadratic Heat Pipe : Subsystem
      mask Display:
      | plot([-1:0.2:1], [1 .7 .5 .4 .35 .32 .35 .4 .5 .7 1])
      | plot([-1:0.2:1], -[1 .7 .5 .4 .35 .32 .35 .4 .5 .7 1])
  Quadratic Pipe : Subsystem
      mask Display:
      | plot([-1:0.2:1], [1 .7 .5 .4 .35 .32 .35 .4 .5 .7 1])
      | plot([-1:0.2:1], -[1 .7 .5 .4 .35 .32 .35 .4 .5 .7 1])
  Tank : Subsystem
      mask Display:
      | color('white')
      | plot([-1 1 1 -1 -1], [-1 -1 1 1 -1])
      | 
      | color('black')
      | plot([1.0 1.18 1.18 1.0], [0 .15 -.15 0])
      | 
      | plot([-0.4 -0.4],[-1 1])
      | plot([-0.4 0], [-1 -1])
      | plot([-0.4 0],[1 1])
      | 
      | plot([-0.3 1],[0 0])
  Water-Glycol Heat Exchanger : Subsystem
  X Heat Exchanger : Subsystem

== system Simple_lib/Junkyard ==
  CinWall : Subsystem  AncestorBlock=PlantUtilityBlockset_lib/Electrical/C0
      mask Display:
      | color('white')
      | plot([-1 1 1 -1 -1], [-1 -1 1 1 -1])
      | 
      | color('red')
      | plot([1.0 1.18 1.18 1.0], [0 .15 -.15 0])
      | patch([1.0 1.0 0.8 0.8 0.7 -0.9 -1.0 -1.0 -0.9  0.7  0.8 0.8   1.0 1.0],        [0.0 0.3 0.2 0.9 1.0 1.0   0.9 -0.9 -1.0 -1.0 -0.9 -0.2 -0.3 0.0],       [.8 0 0])
  "Conventional Flow " : Subsystem
      mask Display:
      | color('white')
      | plot([-1 -1], [-2 2])
      | plot([1 1], [-2 2])
      | color('black')
      | plot(-[1 0 0 -1 -1 0 0 1], [0 2 1 1 -1 -1 -2 0])
  R13 : Subsystem  AncestorBlock=PlantUtilityBlockset_lib/Electrical/R  mask{R=1/wallArea/h_A_W}
      mask prompts: R "Resistance"
      mask Display:
      | color('white')
      | plot([-1 1 1 -1 -1], [-1 -1 1 1 -1])
      | color('red')
      | plot([1.0 1.18 1.18 1.0], [0 .2 -.2 0])
      | plot([1 1],[-1 1])
      | plot([-8:8]/8, cos([-8:8])/2)
  R17 : Subsystem  AncestorBlock=PlantUtilityBlockset_lib/Electrical/R1  mask{R=LWall/kWall/wallArea/2}
      mask prompts: R "Resistance"
      mask Display:
      | color('white')
      | plot([-1 1 1 -1 -1], [-1 -1 1 1 -1])
      | color('red')
      | patch( [ -1 1 1 -1 -1],[-.51 -.51  -.49 -.49 -.51],[0.85 0 0])
      | patch( [ -1 1 1 -1 -1],[ .51  .51   .49  .49  .51],[0.85 0 0])
      | plot( [ .6 1],[-.5 .2])
      | plot( [ .3 .8],[-.5 .5])
      | plot( [ .0 .5],[-.5 .5])
      | plot( [-.3 .2],[-.5 .5])
      | plot( [-.6 -.1],[-.5 .5])
      | plot( [-.9 -.4],[-.5 .5])
      | plot( [-1 -.7],[-.1 .5])
      | %plot( [ -1 0 1 0 -1 0 1 0 -1 0 1 0 -1],[-6:6]/12)
  ThermoMeter : Subsystem
      mask Display:
      | color('white')
      | plot([-1 1 1 -1 -1], [-1 -1 1 1 -1])
      | color('black')
      | 
      | plot([-1 -.9 -.5 0 .5 .9 1  .9  .5  0 -.5 -.9 -1], ...
      |     [ 0  .5 .9 1 .9 .5 0 -.5 -.9 -1 -.9 -.5  0]);
      | plot(.7*[-1 1], .7*[-1 1])
      | plot(.7*[-1 1], .7*[1 -1])
      | 
      | %text(0, 0, 'p')
  Unconventional Flow : Subsystem
      mask Display:
      | color('white')
      | plot([-1 -1], [2 2])
      | plot([1 1], [-2 -2])
      | color('black')
      | plot([1 0 0 -1 -1 0 0 1], [0 2 1 1 -1 -1 -2 0])
